simulink model "ovap_sim"  (R2025a)
settings: Solver=ode4  StartTime=0.0  StopTime=20  FixedStep=0.002  RelTol=1e-3
undefined symbols (not defined in the file): X, Y, Z
libraries: sm_lib x173, nesl_utility x72, simulink_extras x37, slpidlib x16, fl_lib x2
(part 4 of 5)

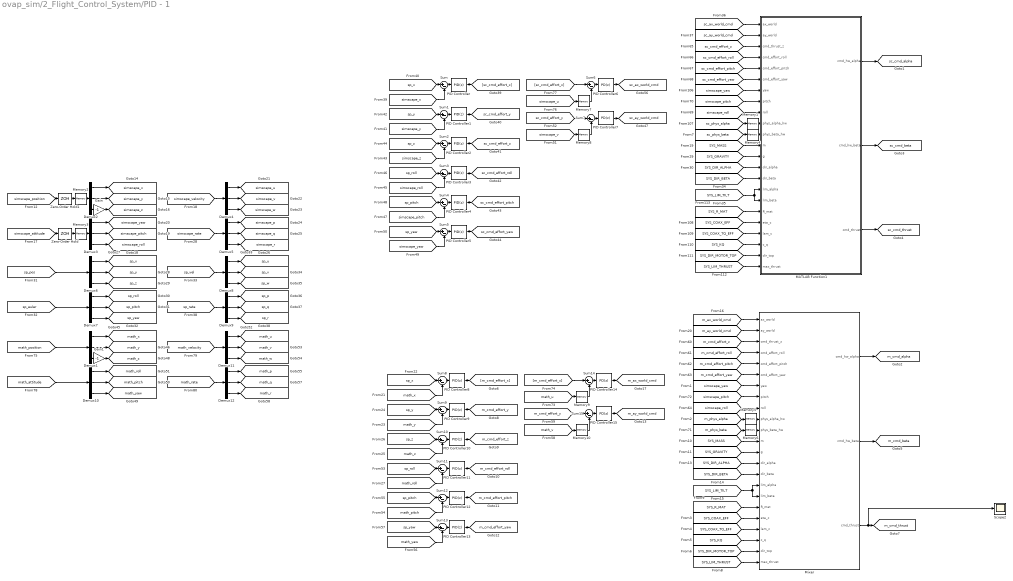
== system ovap_sim/2_Flight_Control_System/PID - 1 ==
  Demux{1..12} (12 alike) : Demux  Outputs=3
  Gain : Gain  Gain=-1
  Gain1 : Gain  Gain=-1
  MATLAB Function1 : MATLAB Function  TreatAsAtomicUnit=on
  Memory{1..10} (10 alike) : Memory
  Mixer : MATLAB Function  TreatAsAtomicUnit=on
  PID Controller : slpidlib/PID Controller  Controller=PID  Form=Parallel  TimeDomain=Discrete-time  UseExternalTs=off  SampleTime=0.002  IntegratorMethod=Forward Euler  FilterMethod=Forward Euler  ControllerParametersSource=internal  P=1  I=0  UseKiTs=off  D=0  UseExternalDerivativeSource=off  N=100  UseFilter=on  TunerSelectOption=Transfer Function Based (PID Tuner App)  InitialConditionSource=internal  InitialConditionForIntegrator=0  InitialConditionForFilter=0  DifferentiatorICPrevScaledInput=0  ExternalReset=none  TrackingMode=off  Kt=1  LimitOutput=off  SatLimitsSource=internal  UpperSaturationLimit=1  LowerSaturationLimit=-1  LinearizeAsGain=off  AntiWindupMode=clamping  Kb=1  LimitIntegrator=off  UpperIntegratorSaturationLimit=inf  LowerIntegratorSaturationLimit=-inf  POutMin=[]  POutMax=[]  IOutMin=[]  IOutMax=[]  DOutMin=[]  DOutMax=[]  NOutMin=[]  NOutMax=[]  SumOutMin=[]  SumOutMax=[]  SaturationOutMin=[]  SaturationOutMax=[]  PParamMin=[]  PParamMax=[]  IParamMin=[]  IParamMax=[]  DParamMin=[]  DParamMax=[]  NParamMin=[]  NParamMax=[]  KbParamMin=[]  KbParamMax=[]  KtParamMin=[]  KtParamMax=[]  KbOutMin=[]  KbOutMax=[]  KtOutMin=[]  KtOutMax=[]  IntegratorOutMin=[]  IntegratorOutMax=[]  FilterOutMin=[]  FilterOutMax=[]  SumI1OutMin=[]  SumI1OutMax=[]  SumI2OutMin=[]  SumI2OutMax=[]  SumI3OutMin=[]  SumI3OutMax=[]  SumI4OutMin=[]  SumI4OutMax=[]  SumDOutMin=[]  SumDOutMax=[]  DifferentiatorOutMin=[]  DifferentiatorOutMax=[]  FilterDiffOutCoefMin=[]  FilterDiffOutCoefMax=[]  ReciprocalOutMin=[]  ReciprocalOutMax=[]  SumDenOutMin=[]  SumDenOutMax=[]  SumNumOutMin=[]  SumNumOutMax=[]  DivideOutMin=[]  DivideOutMax=[]  UdiffTsProdOutMin=[]  UdiffTsProdOutMax=[]  NTsProdOutMin=[]  NTsProdOutMax=[]  UintegralTsProdOutMin=[]  UintegralTsProdOutMax=[]  UngainTsProdOutMin=[]  UngainTsProdOutMax=[]  ClampingZeroOutDataTypeStr=Inherit: Inherit via back propagation  ClampingZeroOutMin=[]  ClampingZeroOutMax=[]  FilterDenConstantOutDataTypeStr=Inherit: Inherit via back propagation  FilterDenConstantOutMin=[]  FilterDenConstantOutMax=[]  PCopyOutDataTypeStr=Inherit: Inherit via back propagation  PCopyOutMin=[]  PCopyOutMax=[]  NCopyOutDataTypeStr=Inherit: Inherit via back propagation  NCopyOutMin=[]  NCopyOutMax=[]  IntegratorContinuousStateAttributes=''  IntegratorStateMustResolveToSignalObject=off  IntegratorRTWStateStorageClass=Auto  FilterContinuousStateAttributes=''  FilterStateMustResolveToSignalObject=off  FilterRTWStateStorageClass=Auto  ParallelPVariant=InternalParameters  IdealPVariant=Disabled  IVariant=InternalParameters  DVariant=InternalParameters  IntegratorVariant=Discrete  SatVariant=Disabled  AWVariant=Passthrough  PCopyVariant=Disabled  TRVariant=Disabled  FdbkBlocksVariant=Forward  IdealPFdbkVariant=Disabled  SatFdbkVariant=Disabled  DerivativeFilterVariant=ForwardEulerFilter  NVariant=InternalParameters  NCopyVariant=Disabled  FilterICVariant=InternalICsFilter  IntegratorICVariant=InternalICs  ExternalResetVariant=Disabled  TRSumVariant=Passthrough  SumFdbkVariant=Disabled  SumVariant=Sum_PID  TsampFilterVariant=InternalTs  TsampNgainVariant=Passthrough  TsampIntegralVariant=Disabled_SignalSpec  ExternalSaturationOutDataTypeStr=Inherit: Same as second input  DerivativeSourceVariant=ErrorSignal  PreIntVariant=InternalPreInt
  PID Controller1 : slpidlib/PID Controller  Controller=PID  Form=Parallel  TimeDomain=Discrete-time  UseExternalTs=off  SampleTime=0.002  IntegratorMethod=Forward Euler  FilterMethod=Forward Euler  ControllerParametersSource=internal  P=1  I=0  UseKiTs=off  D=0  UseExternalDerivativeSource=off  N=100  UseFilter=on  TunerSelectOption=Transfer Function Based (PID Tuner App)  InitialConditionSource=internal  InitialConditionForIntegrator=0  InitialConditionForFilter=0  DifferentiatorICPrevScaledInput=0  ExternalReset=none  TrackingMode=off  Kt=1  LimitOutput=on  SatLimitsSource=internal  UpperSaturationLimit=5  LowerSaturationLimit=-5  LinearizeAsGain=on  AntiWindupMode=clamping  Kb=1  LimitIntegrator=off  UpperIntegratorSaturationLimit=inf  LowerIntegratorSaturationLimit=-inf  POutMin=[]  POutMax=[]  IOutMin=[]  IOutMax=[]  DOutMin=[]  DOutMax=[]  NOutMin=[]  NOutMax=[]  SumOutMin=[]  SumOutMax=[]  SaturationOutMin=[]  SaturationOutMax=[]  PParamMin=[]  PParamMax=[]  IParamMin=[]  IParamMax=[]  DParamMin=[]  DParamMax=[]  NParamMin=[]  NParamMax=[]  KbParamMin=[]  KbParamMax=[]  KtParamMin=[]  KtParamMax=[]  KbOutMin=[]  KbOutMax=[]  KtOutMin=[]  KtOutMax=[]  IntegratorOutMin=[]  IntegratorOutMax=[]  FilterOutMin=[]  FilterOutMax=[]  SumI1OutMin=[]  SumI1OutMax=[]  SumI2OutMin=[]  SumI2OutMax=[]  SumI3OutMin=[]  SumI3OutMax=[]  SumI4OutMin=[]  SumI4OutMax=[]  SumDOutMin=[]  SumDOutMax=[]  DifferentiatorOutMin=[]  DifferentiatorOutMax=[]  FilterDiffOutCoefMin=[]  FilterDiffOutCoefMax=[]  ReciprocalOutMin=[]  ReciprocalOutMax=[]  SumDenOutMin=[]  SumDenOutMax=[]  SumNumOutMin=[]  SumNumOutMax=[]  DivideOutMin=[]  DivideOutMax=[]  UdiffTsProdOutMin=[]  UdiffTsProdOutMax=[]  NTsProdOutMin=[]  NTsProdOutMax=[]  UintegralTsProdOutMin=[]  UintegralTsProdOutMax=[]  UngainTsProdOutMin=[]  UngainTsProdOutMax=[]  ClampingZeroOutDataTypeStr=Inherit: Inherit via back propagation  ClampingZeroOutMin=[]  ClampingZeroOutMax=[]  FilterDenConstantOutDataTypeStr=Inherit: Inherit via back propagation  FilterDenConstantOutMin=[]  FilterDenConstantOutMax=[]  PCopyOutDataTypeStr=Inherit: Inherit via back propagation  PCopyOutMin=[]  PCopyOutMax=[]  NCopyOutDataTypeStr=Inherit: Inherit via back propagation  NCopyOutMin=[]  NCopyOutMax=[]  IntegratorContinuousStateAttributes=''  IntegratorStateMustResolveToSignalObject=off  IntegratorRTWStateStorageClass=Auto  FilterContinuousStateAttributes=''  FilterStateMustResolveToSignalObject=off  FilterRTWStateStorageClass=Auto  ParallelPVariant=InternalParameters  IdealPVariant=Disabled  IVariant=InternalParameters  DVariant=InternalParameters  IntegratorVariant=Discrete  SatVariant=Enabled  AWVariant=DiscClampingParallel  PCopyVariant=Disabled  TRVariant=Disabled  FdbkBlocksVariant=Forward  IdealPFdbkVariant=Disabled  SatFdbkVariant=Disabled  DerivativeFilterVariant=ForwardEulerFilter  NVariant=InternalParameters  NCopyVariant=Disabled  FilterICVariant=InternalICsFilter  IntegratorICVariant=InternalICs  ExternalResetVariant=Disabled  TRSumVariant=Passthrough  SumFdbkVariant=Disabled  SumVariant=Sum_PID  TsampFilterVariant=InternalTs  TsampNgainVariant=Passthrough  TsampIntegralVariant=Disabled_SignalSpec  ExternalSaturationOutDataTypeStr=Inherit: Same as second input  DerivativeSourceVariant=ErrorSignal  PreIntVariant=InternalPreInt
  PID Controller10 : slpidlib/PID Controller  Controller=PID  Form=Parallel  TimeDomain=Discrete-time  UseExternalTs=off  SampleTime=0.002  IntegratorMethod=Forward Euler  FilterMethod=Forward Euler  ControllerParametersSource=internal  P=2  I=0.0001  UseKiTs=off  D=4  UseExternalDerivativeSource=off  N=100  UseFilter=on  TunerSelectOption=Transfer Function Based (PID Tuner App)  InitialConditionSource=internal  InitialConditionForIntegrator=0  InitialConditionForFilter=0  DifferentiatorICPrevScaledInput=0  ExternalReset=none  TrackingMode=off  Kt=1  LimitOutput=on  SatLimitsSource=internal  UpperSaturationLimit=5  LowerSaturationLimit=-5  LinearizeAsGain=on  AntiWindupMode=clamping  Kb=1  LimitIntegrator=off  UpperIntegratorSaturationLimit=inf  LowerIntegratorSaturationLimit=-inf  POutMin=[]  POutMax=[]  IOutMin=[]  IOutMax=[]  DOutMin=[]  DOutMax=[]  NOutMin=[]  NOutMax=[]  SumOutMin=[]  SumOutMax=[]  SaturationOutMin=[]  SaturationOutMax=[]  PParamMin=[]  PParamMax=[]  IParamMin=[]  IParamMax=[]  DParamMin=[]  DParamMax=[]  NParamMin=[]  NParamMax=[]  KbParamMin=[]  KbParamMax=[]  KtParamMin=[]  KtParamMax=[]  KbOutMin=[]  KbOutMax=[]  KtOutMin=[]  KtOutMax=[]  IntegratorOutMin=[]  IntegratorOutMax=[]  FilterOutMin=[]  FilterOutMax=[]  SumI1OutMin=[]  SumI1OutMax=[]  SumI2OutMin=[]  SumI2OutMax=[]  SumI3OutMin=[]  SumI3OutMax=[]  SumI4OutMin=[]  SumI4OutMax=[]  SumDOutMin=[]  SumDOutMax=[]  DifferentiatorOutMin=[]  DifferentiatorOutMax=[]  FilterDiffOutCoefMin=[]  FilterDiffOutCoefMax=[]  ReciprocalOutMin=[]  ReciprocalOutMax=[]  SumDenOutMin=[]  SumDenOutMax=[]  SumNumOutMin=[]  SumNumOutMax=[]  DivideOutMin=[]  DivideOutMax=[]  UdiffTsProdOutMin=[]  UdiffTsProdOutMax=[]  NTsProdOutMin=[]  NTsProdOutMax=[]  UintegralTsProdOutMin=[]  UintegralTsProdOutMax=[]  UngainTsProdOutMin=[]  UngainTsProdOutMax=[]  ClampingZeroOutDataTypeStr=Inherit: Inherit via back propagation  ClampingZeroOutMin=[]  ClampingZeroOutMax=[]  FilterDenConstantOutDataTypeStr=Inherit: Inherit via back propagation  FilterDenConstantOutMin=[]  FilterDenConstantOutMax=[]  PCopyOutDataTypeStr=Inherit: Inherit via back propagation  PCopyOutMin=[]  PCopyOutMax=[]  NCopyOutDataTypeStr=Inherit: Inherit via back propagation  NCopyOutMin=[]  NCopyOutMax=[]  IntegratorContinuousStateAttributes=''  IntegratorStateMustResolveToSignalObject=off  IntegratorRTWStateStorageClass=Auto  FilterContinuousStateAttributes=''  FilterStateMustResolveToSignalObject=off  FilterRTWStateStorageClass=Auto  ParallelPVariant=InternalParameters  IdealPVariant=Disabled  IVariant=InternalParameters  DVariant=InternalParameters  IntegratorVariant=Discrete  SatVariant=Enabled  AWVariant=DiscClampingParallel  PCopyVariant=Disabled  TRVariant=Disabled  FdbkBlocksVariant=Forward  IdealPFdbkVariant=Disabled  SatFdbkVariant=Disabled  DerivativeFilterVariant=ForwardEulerFilter  NVariant=InternalParameters  NCopyVariant=Disabled  FilterICVariant=InternalICsFilter  IntegratorICVariant=InternalICs  ExternalResetVariant=Disabled  TRSumVariant=Passthrough  SumFdbkVariant=Disabled  SumVariant=Sum_PID  TsampFilterVariant=InternalTs  TsampNgainVariant=Passthrough  TsampIntegralVariant=Disabled_SignalSpec  ExternalSaturationOutDataTypeStr=Inherit: Same as second input  DerivativeSourceVariant=ErrorSignal  PreIntVariant=InternalPreInt
  PID Controller{3..5,11..13} (6 alike) : slpidlib/PID Controller  Controller=PID  Form=Parallel  TimeDomain=Discrete-time  UseExternalTs=off  SampleTime=0.002  IntegratorMethod=Forward Euler  FilterMethod=Forward Euler  ControllerParametersSource=internal  P=1  I=0  UseKiTs=off  D=0  UseExternalDerivativeSource=off  N=100  UseFilter=on  TunerSelectOption=Transfer Function Based (PID Tuner App)  InitialConditionSource=internal  InitialConditionForIntegrator=0  InitialConditionForFilter=0  DifferentiatorICPrevScaledInput=0  ExternalReset=none  TrackingMode=off  Kt=1  LimitOutput=on  SatLimitsSource=internal  UpperSaturationLimit=5  LowerSaturationLimit=-5  LinearizeAsGain=on  AntiWindupMode=none  Kb=1  LimitIntegrator=off  UpperIntegratorSaturationLimit=inf  LowerIntegratorSaturationLimit=-inf  POutMin=[]  POutMax=[]  IOutMin=[]  IOutMax=[]  DOutMin=[]  DOutMax=[]  NOutMin=[]  NOutMax=[]  SumOutMin=[]  SumOutMax=[]  SaturationOutMin=[]  SaturationOutMax=[]  PParamMin=[]  PParamMax=[]  IParamMin=[]  IParamMax=[]  DParamMin=[]  DParamMax=[]  NParamMin=[]  NParamMax=[]  KbParamMin=[]  KbParamMax=[]  KtParamMin=[]  KtParamMax=[]  KbOutMin=[]  KbOutMax=[]  KtOutMin=[]  KtOutMax=[]  IntegratorOutMin=[]  IntegratorOutMax=[]  FilterOutMin=[]  FilterOutMax=[]  SumI1OutMin=[]  SumI1OutMax=[]  SumI2OutMin=[]  SumI2OutMax=[]  SumI3OutMin=[]  SumI3OutMax=[]  SumI4OutMin=[]  SumI4OutMax=[]  SumDOutMin=[]  SumDOutMax=[]  DifferentiatorOutMin=[]  DifferentiatorOutMax=[]  FilterDiffOutCoefMin=[]  FilterDiffOutCoefMax=[]  ReciprocalOutMin=[]  ReciprocalOutMax=[]  SumDenOutMin=[]  SumDenOutMax=[]  SumNumOutMin=[]  SumNumOutMax=[]  DivideOutMin=[]  DivideOutMax=[]  UdiffTsProdOutMin=[]  UdiffTsProdOutMax=[]  NTsProdOutMin=[]  NTsProdOutMax=[]  UintegralTsProdOutMin=[]  UintegralTsProdOutMax=[]  UngainTsProdOutMin=[]  UngainTsProdOutMax=[]  ClampingZeroOutDataTypeStr=Inherit: Inherit via back propagation  ClampingZeroOutMin=[]  ClampingZeroOutMax=[]  FilterDenConstantOutDataTypeStr=Inherit: Inherit via back propagation  FilterDenConstantOutMin=[]  FilterDenConstantOutMax=[]  PCopyOutDataTypeStr=Inherit: Inherit via back propagation  PCopyOutMin=[]  PCopyOutMax=[]  NCopyOutDataTypeStr=Inherit: Inherit via back propagation  NCopyOutMin=[]  NCopyOutMax=[]  IntegratorContinuousStateAttributes=''  IntegratorStateMustResolveToSignalObject=off  IntegratorRTWStateStorageClass=Auto  FilterContinuousStateAttributes=''  FilterStateMustResolveToSignalObject=off  FilterRTWStateStorageClass=Auto  ParallelPVariant=InternalParameters  IdealPVariant=Disabled  IVariant=InternalParameters  DVariant=InternalParameters  IntegratorVariant=Discrete  SatVariant=Enabled  AWVariant=Passthrough  PCopyVariant=Disabled  TRVariant=Disabled  FdbkBlocksVariant=Forward  IdealPFdbkVariant=Disabled  SatFdbkVariant=Disabled  DerivativeFilterVariant=ForwardEulerFilter  NVariant=InternalParameters  NCopyVariant=Disabled  FilterICVariant=InternalICsFilter  IntegratorICVariant=InternalICs  ExternalResetVariant=Disabled  TRSumVariant=Passthrough  SumFdbkVariant=Disabled  SumVariant=Sum_PID  TsampFilterVariant=InternalTs  TsampNgainVariant=Passthrough  TsampIntegralVariant=Disabled_SignalSpec  ExternalSaturationOutDataTypeStr=Inherit: Same as second input  DerivativeSourceVariant=ErrorSignal  PreIntVariant=InternalPreInt
  PID Controller{6..7,14..15} (4 alike) : slpidlib/PID Controller  Controller=PD  Form=Parallel  TimeDomain=Discrete-time  UseExternalTs=off  SampleTime=0.002  IntegratorMethod=Forward Euler  FilterMethod=Forward Euler  ControllerParametersSource=internal  P=1  I=0  UseKiTs=off  D=0  UseExternalDerivativeSource=off  N=100  UseFilter=on  TunerSelectOption=Transfer Function Based (PID Tuner App)  InitialConditionSource=internal  InitialConditionForIntegrator=0  InitialConditionForFilter=0  DifferentiatorICPrevScaledInput=0  ExternalReset=none  TrackingMode=off  Kt=1  LimitOutput=on  SatLimitsSource=internal  UpperSaturationLimit=3  LowerSaturationLimit=-3  LinearizeAsGain=off  AntiWindupMode=clamping  Kb=1  LimitIntegrator=off  UpperIntegratorSaturationLimit=inf  LowerIntegratorSaturationLimit=-inf  POutMin=[]  POutMax=[]  IOutMin=[]  IOutMax=[]  DOutMin=[]  DOutMax=[]  NOutMin=[]  NOutMax=[]  SumOutMin=[]  SumOutMax=[]  SaturationOutMin=[]  SaturationOutMax=[]  PParamMin=[]  PParamMax=[]  IParamMin=[]  IParamMax=[]  DParamMin=[]  DParamMax=[]  NParamMin=[]  NParamMax=[]  KbParamMin=[]  KbParamMax=[]  KtParamMin=[]  KtParamMax=[]  KbOutMin=[]  KbOutMax=[]  KtOutMin=[]  KtOutMax=[]  IntegratorOutMin=[]  IntegratorOutMax=[]  FilterOutMin=[]  FilterOutMax=[]  SumI1OutMin=[]  SumI1OutMax=[]  SumI2OutMin=[]  SumI2OutMax=[]  SumI3OutMin=[]  SumI3OutMax=[]  SumI4OutMin=[]  SumI4OutMax=[]  SumDOutMin=[]  SumDOutMax=[]  DifferentiatorOutMin=[]  DifferentiatorOutMax=[]  FilterDiffOutCoefMin=[]  FilterDiffOutCoefMax=[]  ReciprocalOutMin=[]  ReciprocalOutMax=[]  SumDenOutMin=[]  SumDenOutMax=[]  SumNumOutMin=[]  SumNumOutMax=[]  DivideOutMin=[]  DivideOutMax=[]  UdiffTsProdOutMin=[]  UdiffTsProdOutMax=[]  NTsProdOutMin=[]  NTsProdOutMax=[]  UintegralTsProdOutMin=[]  UintegralTsProdOutMax=[]  UngainTsProdOutMin=[]  UngainTsProdOutMax=[]  ClampingZeroOutDataTypeStr=Inherit: Inherit via back propagation  ClampingZeroOutMin=[]  ClampingZeroOutMax=[]  FilterDenConstantOutDataTypeStr=Inherit: Inherit via back propagation  FilterDenConstantOutMin=[]  FilterDenConstantOutMax=[]  PCopyOutDataTypeStr=Inherit: Inherit via back propagation  PCopyOutMin=[]  PCopyOutMax=[]  NCopyOutDataTypeStr=Inherit: Inherit via back propagation  NCopyOutMin=[]  NCopyOutMax=[]  IntegratorContinuousStateAttributes=''  IntegratorStateMustResolveToSignalObject=off  IntegratorRTWStateStorageClass=Auto  FilterContinuousStateAttributes=''  FilterStateMustResolveToSignalObject=off  FilterRTWStateStorageClass=Auto  ParallelPVariant=InternalParameters  IdealPVariant=Disabled  IVariant=Disabled  DVariant=InternalParameters  IntegratorVariant=Disabled  SatVariant=Enabled  AWVariant=Disabled  PCopyVariant=Disabled  TRVariant=Disabled  FdbkBlocksVariant=Forward  IdealPFdbkVariant=Disabled  SatFdbkVariant=Disabled  DerivativeFilterVariant=ForwardEulerFilter  NVariant=InternalParameters  NCopyVariant=Disabled  FilterICVariant=InternalICsFilter  IntegratorICVariant=Disabled  ExternalResetVariant=Disabled  TRSumVariant=Passthrough  SumFdbkVariant=Disabled  SumVariant=Sum_PD  TsampFilterVariant=InternalTs  TsampNgainVariant=Passthrough  TsampIntegralVariant=Disabled_SignalSpec  ExternalSaturationOutDataTypeStr=Inherit: Same as second input  DerivativeSourceVariant=ErrorSignal  PreIntVariant=InternalPreInt
  PID Controller2 : slpidlib/PID Controller  Controller=PID  Form=Parallel  TimeDomain=Discrete-time  UseExternalTs=off  SampleTime=0.002  IntegratorMethod=Forward Euler  FilterMethod=Forward Euler  ControllerParametersSource=internal  P=2  I=0.0001  UseKiTs=off  D=4.2  UseExternalDerivativeSource=off  N=100  UseFilter=on  TunerSelectOption=Transfer Function Based (PID Tuner App)  InitialConditionSource=internal  InitialConditionForIntegrator=0  InitialConditionForFilter=0  DifferentiatorICPrevScaledInput=0  ExternalReset=none  TrackingMode=off  Kt=1  LimitOutput=on  SatLimitsSource=internal  UpperSaturationLimit=5  LowerSaturationLimit=-5  LinearizeAsGain=on  AntiWindupMode=clamping  Kb=1  LimitIntegrator=off  UpperIntegratorSaturationLimit=inf  LowerIntegratorSaturationLimit=-inf  POutMin=[]  POutMax=[]  IOutMin=[]  IOutMax=[]  DOutMin=[]  DOutMax=[]  NOutMin=[]  NOutMax=[]  SumOutMin=[]  SumOutMax=[]  SaturationOutMin=[]  SaturationOutMax=[]  PParamMin=[]  PParamMax=[]  IParamMin=[]  IParamMax=[]  DParamMin=[]  DParamMax=[]  NParamMin=[]  NParamMax=[]  KbParamMin=[]  KbParamMax=[]  KtParamMin=[]  KtParamMax=[]  KbOutMin=[]  KbOutMax=[]  KtOutMin=[]  KtOutMax=[]  IntegratorOutMin=[]  IntegratorOutMax=[]  FilterOutMin=[]  FilterOutMax=[]  SumI1OutMin=[]  SumI1OutMax=[]  SumI2OutMin=[]  SumI2OutMax=[]  SumI3OutMin=[]  SumI3OutMax=[]  SumI4OutMin=[]  SumI4OutMax=[]  SumDOutMin=[]  SumDOutMax=[]  DifferentiatorOutMin=[]  DifferentiatorOutMax=[]  FilterDiffOutCoefMin=[]  FilterDiffOutCoefMax=[]  ReciprocalOutMin=[]  ReciprocalOutMax=[]  SumDenOutMin=[]  SumDenOutMax=[]  SumNumOutMin=[]  SumNumOutMax=[]  DivideOutMin=[]  DivideOutMax=[]  UdiffTsProdOutMin=[]  UdiffTsProdOutMax=[]  NTsProdOutMin=[]  NTsProdOutMax=[]  UintegralTsProdOutMin=[]  UintegralTsProdOutMax=[]  UngainTsProdOutMin=[]  UngainTsProdOutMax=[]  ClampingZeroOutDataTypeStr=Inherit: Inherit via back propagation  ClampingZeroOutMin=[]  ClampingZeroOutMax=[]  FilterDenConstantOutDataTypeStr=Inherit: Inherit via back propagation  FilterDenConstantOutMin=[]  FilterDenConstantOutMax=[]  PCopyOutDataTypeStr=Inherit: Inherit via back propagation  PCopyOutMin=[]  PCopyOutMax=[]  NCopyOutDataTypeStr=Inherit: Inherit via back propagation  NCopyOutMin=[]  NCopyOutMax=[]  IntegratorContinuousStateAttributes=''  IntegratorStateMustResolveToSignalObject=off  IntegratorRTWStateStorageClass=Auto  FilterContinuousStateAttributes=''  FilterStateMustResolveToSignalObject=off  FilterRTWStateStorageClass=Auto  ParallelPVariant=InternalParameters  IdealPVariant=Disabled  IVariant=InternalParameters  DVariant=InternalParameters  IntegratorVariant=Discrete  SatVariant=Enabled  AWVariant=DiscClampingParallel  PCopyVariant=Disabled  TRVariant=Disabled  FdbkBlocksVariant=Forward  IdealPFdbkVariant=Disabled  SatFdbkVariant=Disabled  DerivativeFilterVariant=ForwardEulerFilter  NVariant=InternalParameters  NCopyVariant=Disabled  FilterICVariant=InternalICsFilter  IntegratorICVariant=InternalICs  ExternalResetVariant=Disabled  TRSumVariant=Passthrough  SumFdbkVariant=Disabled  SumVariant=Sum_PID  TsampFilterVariant=InternalTs  TsampNgainVariant=Passthrough  TsampIntegralVariant=Disabled_SignalSpec  ExternalSaturationOutDataTypeStr=Inherit: Same as second input  DerivativeSourceVariant=ErrorSignal  PreIntVariant=InternalPreInt
  PID Controller8 : slpidlib/PID Controller  Controller=PID  Form=Parallel  TimeDomain=Discrete-time  UseExternalTs=off  SampleTime=0.002  IntegratorMethod=Forward Euler  FilterMethod=Forward Euler  ControllerParametersSource=internal  P=1  I=0  UseKiTs=off  D=0  UseExternalDerivativeSource=off  N=100  UseFilter=on  TunerSelectOption=Transfer Function Based (PID Tuner App)  InitialConditionSource=internal  InitialConditionForIntegrator=0  InitialConditionForFilter=0  DifferentiatorICPrevScaledInput=0  ExternalReset=none  TrackingMode=off  Kt=1  LimitOutput=off  SatLimitsSource=internal  UpperSaturationLimit=1  LowerSaturationLimit=-1  LinearizeAsGain=off  AntiWindupMode=clamping  Kb=1  LimitIntegrator=off  UpperIntegratorSaturationLimit=inf  LowerIntegratorSaturationLimit=-inf  POutMin=[]  POutMax=[]  IOutMin=[]  IOutMax=[]  DOutMin=[]  DOutMax=[]  NOutMin=[]  NOutMax=[]  SumOutMin=[]  SumOutMax=[]  SaturationOutMin=[]  SaturationOutMax=[]  PParamMin=[]  PParamMax=[]  IParamMin=[]  IParamMax=[]  DParamMin=[]  DParamMax=[]  NParamMin=[]  NParamMax=[]  KbParamMin=[]  KbParamMax=[]  KtParamMin=[]  KtParamMax=[]  KbOutMin=[]  KbOutMax=[]  KtOutMin=[]  KtOutMax=[]  IntegratorOutMin=[]  IntegratorOutMax=[]  FilterOutMin=[]  FilterOutMax=[]  SumI1OutMin=[]  SumI1OutMax=[]  SumI2OutMin=[]  SumI2OutMax=[]  SumI3OutMin=[]  SumI3OutMax=[]  SumI4OutMin=[]  SumI4OutMax=[]  SumDOutMin=[]  SumDOutMax=[]  DifferentiatorOutMin=[]  DifferentiatorOutMax=[]  FilterDiffOutCoefMin=[]  FilterDiffOutCoefMax=[]  ReciprocalOutMin=[]  ReciprocalOutMax=[]  SumDenOutMin=[]  SumDenOutMax=[]  SumNumOutMin=[]  SumNumOutMax=[]  DivideOutMin=[]  DivideOutMax=[]  UdiffTsProdOutMin=[]  UdiffTsProdOutMax=[]  NTsProdOutMin=[]  NTsProdOutMax=[]  UintegralTsProdOutMin=[]  UintegralTsProdOutMax=[]  UngainTsProdOutMin=[]  UngainTsProdOutMax=[]  ClampingZeroOutDataTypeStr=Inherit: Inherit via back propagation  ClampingZeroOutMin=[]  ClampingZeroOutMax=[]  FilterDenConstantOutDataTypeStr=Inherit: Inherit via back propagation  FilterDenConstantOutMin=[]  FilterDenConstantOutMax=[]  PCopyOutDataTypeStr=Inherit: Inherit via back propagation  PCopyOutMin=[]  PCopyOutMax=[]  NCopyOutDataTypeStr=Inherit: Inherit via back propagation  NCopyOutMin=[]  NCopyOutMax=[]  IntegratorContinuousStateAttributes=''  IntegratorStateMustResolveToSignalObject=off  IntegratorRTWStateStorageClass=Auto  FilterContinuousStateAttributes=''  FilterStateMustResolveToSignalObject=off  FilterRTWStateStorageClass=Auto  ParallelPVariant=InternalParameters  IdealPVariant=Disabled  IVariant=InternalParameters  DVariant=InternalParameters  IntegratorVariant=Discrete  SatVariant=Disabled  AWVariant=Passthrough  PCopyVariant=Disabled  TRVariant=Disabled  FdbkBlocksVariant=Forward  IdealPFdbkVariant=Disabled  SatFdbkVariant=Disabled  DerivativeFilterVariant=ForwardEulerFilter  NVariant=InternalParameters  NCopyVariant=Disabled  FilterICVariant=InternalICsFilter  IntegratorICVariant=InternalICs  ExternalResetVariant=Disabled  TRSumVariant=Passthrough  SumFdbkVariant=Disabled  SumVariant=Sum_PID  TsampFilterVariant=InternalTs  TsampNgainVariant=Passthrough  TsampIntegralVariant=Disabled_SignalSpec  ExternalSaturationOutDataTypeStr=Inherit: Same as second input  DerivativeSourceVariant=ErrorSignal  PreIntVariant=InternalPreInt
  PID Controller9 : slpidlib/PID Controller  Controller=PID  Form=Parallel  TimeDomain=Discrete-time  UseExternalTs=off  SampleTime=0.002  IntegratorMethod=Forward Euler  FilterMethod=Forward Euler  ControllerParametersSource=internal  P=1  I=0  UseKiTs=off  D=0  UseExternalDerivativeSource=off  N=100  UseFilter=on  TunerSelectOption=Transfer Function Based (PID Tuner App)  InitialConditionSource=internal  InitialConditionForIntegrator=0  InitialConditionForFilter=0  DifferentiatorICPrevScaledInput=0  ExternalReset=none  TrackingMode=off  Kt=1  LimitOutput=on  SatLimitsSource=internal  UpperSaturationLimit=5  LowerSaturationLimit=-5  LinearizeAsGain=on  AntiWindupMode=clamping  Kb=1  LimitIntegrator=off  UpperIntegratorSaturationLimit=inf  LowerIntegratorSaturationLimit=-inf  POutMin=[]  POutMax=[]  IOutMin=[]  IOutMax=[]  DOutMin=[]  DOutMax=[]  NOutMin=[]  NOutMax=[]  SumOutMin=[]  SumOutMax=[]  SaturationOutMin=[]  SaturationOutMax=[]  PParamMin=[]  PParamMax=[]  IParamMin=[]  IParamMax=[]  DParamMin=[]  DParamMax=[]  NParamMin=[]  NParamMax=[]  KbParamMin=[]  KbParamMax=[]  KtParamMin=[]  KtParamMax=[]  KbOutMin=[]  KbOutMax=[]  KtOutMin=[]  KtOutMax=[]  IntegratorOutMin=[]  IntegratorOutMax=[]  FilterOutMin=[]  FilterOutMax=[]  SumI1OutMin=[]  SumI1OutMax=[]  SumI2OutMin=[]  SumI2OutMax=[]  SumI3OutMin=[]  SumI3OutMax=[]  SumI4OutMin=[]  SumI4OutMax=[]  SumDOutMin=[]  SumDOutMax=[]  DifferentiatorOutMin=[]  DifferentiatorOutMax=[]  FilterDiffOutCoefMin=[]  FilterDiffOutCoefMax=[]  ReciprocalOutMin=[]  ReciprocalOutMax=[]  SumDenOutMin=[]  SumDenOutMax=[]  SumNumOutMin=[]  SumNumOutMax=[]  DivideOutMin=[]  DivideOutMax=[]  UdiffTsProdOutMin=[]  UdiffTsProdOutMax=[]  NTsProdOutMin=[]  NTsProdOutMax=[]  UintegralTsProdOutMin=[]  UintegralTsProdOutMax=[]  UngainTsProdOutMin=[]  UngainTsProdOutMax=[]  ClampingZeroOutDataTypeStr=Inherit: Inherit via back propagation  ClampingZeroOutMin=[]  ClampingZeroOutMax=[]  FilterDenConstantOutDataTypeStr=Inherit: Inherit via back propagation  FilterDenConstantOutMin=[]  FilterDenConstantOutMax=[]  PCopyOutDataTypeStr=Inherit: Inherit via back propagation  PCopyOutMin=[]  PCopyOutMax=[]  NCopyOutDataTypeStr=Inherit: Inherit via back propagation  NCopyOutMin=[]  NCopyOutMax=[]  IntegratorContinuousStateAttributes=''  IntegratorStateMustResolveToSignalObject=off  IntegratorRTWStateStorageClass=Auto  FilterContinuousStateAttributes=''  FilterStateMustResolveToSignalObject=off  FilterRTWStateStorageClass=Auto  ParallelPVariant=InternalParameters  IdealPVariant=Disabled  IVariant=InternalParameters  DVariant=InternalParameters  IntegratorVariant=Discrete  SatVariant=Enabled  AWVariant=DiscClampingParallel  PCopyVariant=Disabled  TRVariant=Disabled  FdbkBlocksVariant=Forward  IdealPFdbkVariant=Disabled  SatFdbkVariant=Disabled  DerivativeFilterVariant=ForwardEulerFilter  NVariant=InternalParameters  NCopyVariant=Disabled  FilterICVariant=InternalICsFilter  IntegratorICVariant=InternalICs  ExternalResetVariant=Disabled  TRSumVariant=Passthrough  SumFdbkVariant=Disabled  SumVariant=Sum_PID  TsampFilterVariant=InternalTs  TsampNgainVariant=Passthrough  TsampIntegralVariant=Disabled_SignalSpec  ExternalSaturationOutDataTypeStr=Inherit: Same as second input  DerivativeSourceVariant=ErrorSignal  PreIntVariant=InternalPreInt
  Scope2 : Scope
      settings: ActiveDisplayYMinimum=2.634685350754407  ActiveDisplayYMaximum=5.63815135293212  DataLoggingVariableName=ScopeData25
  Sum{,1..15} (16 alike) : Sum  Inputs=|+-
  Zero-Order Hold : ZeroOrderHold  SampleTime=0.002
  Zero-Order Hold1 : ZeroOrderHold  SampleTime=0.002
  tag scope: m_ax_world_cmd=global, m_ay_world_cmd=global, m_cmd_alpha=global, m_cmd_beta=global, m_cmd_effort_pitch=global, m_cmd_effort_roll=global, m_cmd_effort_y=global, m_cmd_effort_yaw=global, m_cmd_effort_z=global, m_cmd_thrust=global, math_p=global, math_pitch=global, math_q=global, math_r=global, math_roll=global, math_u=global, math_v=global, math_w=global, math_x=global, math_y=global, math_yaw=global, math_z=global, sc_ax_world_cmd=global, sc_ay_world_cmd=global, sc_cmd_alpha=global, sc_cmd_beta=global, sc_cmd_effort_pitch=global, sc_cmd_effort_roll=global, sc_cmd_effort_y=global, sc_cmd_effort_yaw=global, sc_cmd_effort_z=global, sc_cmd_thrust=global, simscape_p=global, simscape_pitch=global, simscape_q=global, simscape_r=global, simscape_roll=global, simscape_u=global, simscape_v=global, simscape_w=global, simscape_x=global, simscape_y=global, simscape_yaw=global, simscape_z=global, sp_p=global, sp_pitch=global, sp_q=global, sp_r=global, sp_roll=global, sp_u=global, sp_v=global, sp_w=global, sp_x=global, sp_y=global, sp_yaw=global, sp_z=global
  wires:
  [simscape_position] -> Zero-Order Hold1/1
  Demux2/1 -> [simscape_x]
  Demux2/2 -> [simscape_y]
  [simscape_attitude] -> Zero-Order Hold/1
  [simscape_rate] -> Demux5/1
  Demux5/2 -> [simscape_q]
  Demux5/1 -> [simscape_p]
  Demux5/3 -> [simscape_r]
  Demux4/1 -> [simscape_u]
  [simscape_velocity] -> Demux4/1
  Demux4/2 -> [simscape_v]
  Demux4/3 -> [simscape_w]
  Demux7/1 -> [sp_roll]
  Demux7/3 -> [sp_yaw]
  Demux6/1 -> [sp_x]
  [sp_pos] -> Demux6/1
  Demux9/3 -> [sp_r]
  Demux9/1 -> [sp_p]
  Demux9/2 -> [sp_q]
  Demux8/2 -> [sp_v]
  Demux8/3 -> [sp_w]
  Demux8/1 -> [sp_u]
  [sp_vel] -> Demux8/1
  [sp_euler] -> Demux7/1
  Demux7/2 -> [sp_pitch]
  Demux6/2 -> [sp_y]
  Demux6/3 -> [sp_z]
  [sp_rate] -> Demux9/1
  [sp_x] -> Sum/1
  [simscape_x] -> Sum/2
  Sum/1 -> PID Controller/1
  PID Controller/1 -> [sc_cmd_effort_x]
  [simscape_y] -> Sum1/2
  Sum1/1 -> PID Controller1/1
  [sp_y] -> Sum1/1
  PID Controller1/1 -> [sc_cmd_effort_y]
  [simscape_z] -> Sum2/2
  Sum2/1 -> PID Controller2/1
  [sp_z] -> Sum2/1
  PID Controller3/1 -> [sc_cmd_effort_roll]
  [simscape_roll] -> Sum3/2
  PID Controller5/1 -> [sc_cmd_effort_yaw]
  [sp_yaw] -> Sum5/1
  [simscape_yaw] -> Sum5/2
  PID Controller4/1 -> [sc_cmd_effort_pitch]
  [sp_pitch] -> Sum4/1
  Sum4/1 -> PID Controller4/1
  Sum3/1 -> PID Controller3/1
  Sum5/1 -> PID Controller5/1
  [simscape_pitch] -> Sum4/2
  [sp_roll] -> Sum3/1
  Memory2/1 -> Demux2/1
  Memory3/1 -> Demux3/1
  Zero-Order Hold/1 -> Memory3/1
  Zero-Order Hold1/1 -> Memory2/1
  Demux2/3 -> Gain/1
  Gain/1 -> [simscape_z]
  Demux3/1 -> [simscape_yaw]
  Demux3/2 -> [simscape_pitch]
  Demux3/3 -> [simscape_roll]
  Sum6/1 -> PID Controller6/1
  [sc_cmd_effort_x] -> Sum6/1
  [simscape_u] -> Memory7/1
  [simscape_v] -> Memory8/1
  PID Controller7/1 -> [sc_ay_world_cmd]
  [sc_cmd_effort_y] -> Sum7/1
  Sum7/1 -> PID Controller7/1
  Memory7/1 -> Sum6/2
  Memory8/1 -> Sum7/2
  PID Controller6/1 -> [sc_ax_world_cmd]
  MATLAB Function1/1(cmd_hw_alpha) -> [sc_cmd_alpha]
  MATLAB Function1/2(cmd_hw_beta) -> [sc_cmd_beta]
  MATLAB Function1/3(cmd_thrust) -> [sc_cmd_thrust]
  [sc_ax_world_cmd] -> MATLAB Function1/1(ax_world)
  [sc_ay_world_cmd] -> MATLAB Function1/2(ay_world)
  [sc_cmd_effort_z] -> MATLAB Function1/3(cmd_thrust_z)
  [sc_cmd_effort_roll] -> MATLAB Function1/4(cmd_effort_roll)
  [sc_cmd_effort_pitch] -> MATLAB Function1/5(cmd_effort_pitch)
  [sc_cmd_effort_yaw] -> MATLAB Function1/6(cmd_effort_yaw)
  [simscape_yaw] -> MATLAB Function1/7(yaw)
  [simscape_pitch] -> MATLAB Function1/8(pitch)
  [simscape_roll] -> MATLAB Function1/9(roll)
  [SYS_MASS] -> MATLAB Function1/12(m)
  [SYS_GRAVITY] -> MATLAB Function1/13(g)
  [SYS_DIR_ALPHA] -> MATLAB Function1/14(dir_alpha)
  [SYS_DIR_BETA] -> MATLAB Function1/15(dir_beta)
  [SYS_LIM_TILT] -> MATLAB Function1/16(lim_alpha), MATLAB Function1/17(lim_beta)
  [SYS_COAX_EFF] -> MATLAB Function1/19(eta_c)
  [SYS_COAX_TQ_EFF] -> MATLAB Function1/20(lam_c)
  [SYS_KQ] -> MATLAB Function1/21(c_q)
  [SYS_DIR_MOTOR_TOP] -> MATLAB Function1/22(dir_top)
  [SYS_LIM_THRUST] -> MATLAB Function1/23(max_thrust)
  [SYS_R_MAT] -> MATLAB Function1/18(R_mat)
  Memory1/1 -> MATLAB Function1/10(phys_alpha_hw)
  [sc_phys_alpha] -> Memory1/1
  [sc_phys_beta] -> Memory4/1
  Memory4/1 -> MATLAB Function1/11(phys_beta_hw)
  PID Controller2/1 -> [sc_cmd_effort_z]
  [m_cmd_effort_roll] -> Mixer/4(cmd_effort_roll)
  [math_u] -> Memory9/1
  [SYS_LIM_TILT] -> Mixer/16(lim_alpha), Mixer/17(lim_beta)
  [simscape_pitch] -> Mixer/8(pitch)
  [SYS_R_MAT] -> Mixer/18(R_mat)
  Memory10/1 -> Sum15/2
  Sum14/1 -> PID Controller14/1
  [m_cmd_effort_x] -> Sum14/1
  [math_x] -> Sum8/2
  [m_phys_beta] -> Memory6/1
  [math_yaw] -> Sum13/2
  Mixer/2(cmd_hw_beta) -> [m_cmd_beta]
  [sp_yaw] -> Sum13/1
  [SYS_DIR_BETA] -> Mixer/15(dir_beta)
  Mixer/3(cmd_thrust) -> Scope2/1, [m_cmd_thrust]
  Sum10/1 -> PID Controller10/1
  PID Controller11/1 -> [m_cmd_effort_roll]
  [m_cmd_effort_yaw] -> Mixer/6(cmd_effort_yaw)
  PID Controller15/1 -> [m_ay_world_cmd]
  Sum8/1 -> PID Controller8/1
  [SYS_DIR_ALPHA] -> Mixer/14(dir_alpha)
  [sp_y] -> Sum9/1
  Sum15/1 -> PID Controller15/1
  Sum12/1 -> PID Controller12/1
  [m_cmd_effort_y] -> Sum15/1
  [SYS_LIM_THRUST] -> Mixer/23(max_thrust)
  [sp_z] -> Sum10/1
  [m_cmd_effort_z] -> Mixer/3(cmd_thrust_z)
  [SYS_MASS] -> Mixer/12(m)
  PID Controller10/1 -> [m_cmd_effort_z]
  [SYS_DIR_MOTOR_TOP] -> Mixer/22(dir_top)
  PID Controller9/1 -> [m_cmd_effort_y]
  [math_pitch] -> Sum12/2
  PID Controller13/1 -> [m_cmd_effort_yaw]
  [simscape_yaw] -> Mixer/7(yaw)
  [m_ay_world_cmd] -> Mixer/2(ay_world)
  [m_ax_world_cmd] -> Mixer/1(ax_world)
  [SYS_GRAVITY] -> Mixer/13(g)
  Sum11/1 -> PID Controller11/1
  [math_y] -> Sum9/2
  [SYS_COAX_TQ_EFF] -> Mixer/20(lam_c)
  [sp_pitch] -> Sum12/1
  [math_v] -> Memory10/1
  [m_phys_alpha] -> Memory5/1
  [SYS_COAX_EFF] -> Mixer/19(eta_c)
  [sp_roll] -> Sum11/1
  [sp_x] -> Sum8/1
  Memory9/1 -> Sum14/2
  Mixer/1(cmd_hw_alpha) -> [m_cmd_alpha]
  [math_roll] -> Sum11/2
  [simscape_roll] -> Mixer/9(roll)
  [SYS_KQ] -> Mixer/21(c_q)
  [math_z] -> Sum10/2
  Memory6/1 -> Mixer/11(phys_beta_hw)
  PID Controller8/1 -> [m_cmd_effort_x]
  Sum13/1 -> PID Controller13/1
  Memory5/1 -> Mixer/10(phys_alpha_hw)
  PID Controller14/1 -> [m_ax_world_cmd]
  Sum9/1 -> PID Controller9/1
  Demux12/2 -> [math_q]
  [math_attitude] -> Demux10/1
  Demux11/1 -> [math_u]
  Demux11/3 -> [math_w]
  [math_velocity] -> Demux11/1
  Demux10/2 -> [math_pitch]
  Demux12/1 -> [math_p]
  Demux12/3 -> [math_r]
  Demux1/1 -> [math_x]
  Gain1/1 -> [math_z]
  Demux10/1 -> [math_roll]
  [math_rate] -> Demux12/1
  [math_position] -> Demux1/1
  Demux1/2 -> [math_y]
  Demux1/3 -> Gain1/1
  Demux10/3 -> [math_yaw]
  Demux11/2 -> [math_v]
  PID Controller12/1 -> [m_cmd_effort_pitch]
  [m_cmd_effort_pitch] -> Mixer/5(cmd_effort_pitch)

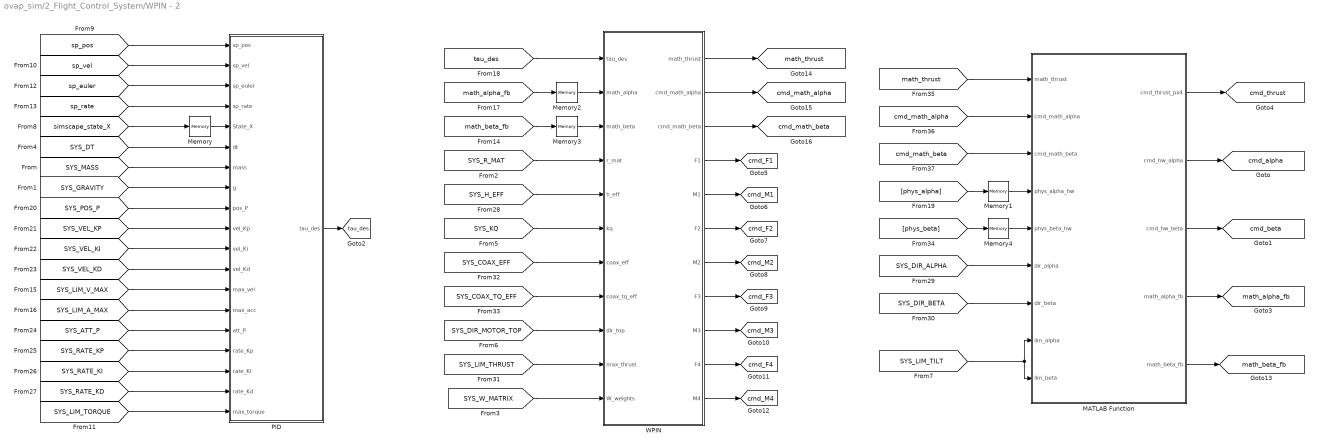
== system ovap_sim/2_Flight_Control_System/WPIN - 2 ==
  MATLAB Function : MATLAB Function  TreatAsAtomicUnit=on
  Memory{,1..4} (5 alike) : Memory
  PID : MATLAB Function  TreatAsAtomicUnit=on
  WPIN : MATLAB Function  TreatAsAtomicUnit=on
  tag scope: cmd_F1=global, cmd_F2=global, cmd_F3=global, cmd_F4=global, cmd_M1=global, cmd_M2=global, cmd_M3=global, cmd_M4=global, cmd_alpha=global, cmd_beta=global, cmd_math_alpha=global, cmd_math_beta=global, cmd_thrust=global, math_alpha_fb=global, math_beta_fb=global, math_thrust=global, tau_des=global
  wires:
  Memory/1 -> PID/5(State_X)
  [SYS_DIR_MOTOR_TOP] -> WPIN/9(dir_top)
  [SYS_RATE_KI] -> PID/17(rate_Ki)
  [SYS_VEL_KP] -> PID/10(vel_Kp)
  [SYS_MASS] -> PID/7(mass)
  [math_beta_fb] -> Memory3/1
  [SYS_LIM_TORQUE] -> PID/19(max_torque)
  [SYS_VEL_KI] -> PID/11(vel_Ki)
  [cmd_math_alpha] -> MATLAB Function/2(cmd_math_alpha)
  MATLAB Function/5(math_beta_fb) -> [math_beta_fb]
  [SYS_GRAVITY] -> PID/8(g)
  Memory4/1 -> MATLAB Function/5(phys_beta_hw)
  [SYS_KQ] -> WPIN/6(kq)
  [phys_alpha] -> Memory1/1
  WPIN/3(cmd_math_beta) -> [cmd_math_beta]
  [SYS_DIR_ALPHA] -> MATLAB Function/6(dir_alpha)
  MATLAB Function/3(cmd_hw_beta) -> [cmd_beta]
  WPIN/1(math_thrust) -> [math_thrust]
  MATLAB Function/2(cmd_hw_alpha) -> [cmd_alpha]
  [SYS_COAX_EFF] -> WPIN/7(coax_eff)
  WPIN/5(M1) -> [cmd_M1]
  [SYS_COAX_TQ_EFF] -> WPIN/8(coax_tq_eff)
  [SYS_H_EFF] -> WPIN/5(h_eff)
  [math_thrust] -> MATLAB Function/1(math_thrust)
  [tau_des] -> WPIN/1(tau_des)
  WPIN/9(M3) -> [cmd_M3]
  [SYS_LIM_THRUST] -> WPIN/10(max_thrust)
  [simscape_state_X] -> Memory/1
  [sp_pos] -> PID/1(sp_pos)
  [SYS_LIM_TILT] -> MATLAB Function/8(lim_alpha), MATLAB Function/9(lim_beta)
  [sp_euler] -> PID/3(sp_euler)
  [cmd_math_beta] -> MATLAB Function/3(cmd_math_beta)
  [SYS_LIM_A_MAX] -> PID/14(max_acc)
  WPIN/11(M4) -> [cmd_M4]
  Memory2/1 -> WPIN/2(math_alpha)
  [SYS_W_MATRIX] -> WPIN/11(W_weights)
  Memory3/1 -> WPIN/3(math_beta)
  WPIN/8(F3) -> [cmd_F3]
  WPIN/10(F4) -> [cmd_F4]
  [sp_vel] -> PID/2(sp_vel)
  WPIN/6(F2) -> [cmd_F2]
  [SYS_RATE_KD] -> PID/18(rate_Kd)
  [SYS_RATE_KP] -> PID/16(rate_Kp)
  [SYS_DT] -> PID/6(dt)
  PID/1(tau_des) -> [tau_des]
  [SYS_VEL_KD] -> PID/12(vel_Kd)
  MATLAB Function/4(math_alpha_fb) -> [math_alpha_fb]
  [phys_beta] -> Memory4/1
  [SYS_POS_P] -> PID/9(pos_P)
  [SYS_DIR_BETA] -> MATLAB Function/7(dir_beta)
  WPIN/7(M2) -> [cmd_M2]
  WPIN/4(F1) -> [cmd_F1]
  [sp_rate] -> PID/4(sp_rate)
  Memory1/1 -> MATLAB Function/4(phys_alpha_hw)
  [SYS_ATT_P] -> PID/15(att_P)
  WPIN/2(cmd_math_alpha) -> [cmd_math_alpha]
  [math_alpha_fb] -> Memory2/1
  [SYS_LIM_V_MAX] -> PID/13(max_vel)
  MATLAB Function/1(cmd_thrust_px4) -> [cmd_thrust]
  [SYS_R_MAT] -> WPIN/4(r_mat)

== matlab function ovap_sim/1_Mission_Planner/MATLAB Function ==
  settings: updateMethod=DISCRETE
  data: t input; dt input; v_max_lim input; a_max_lim input; w_max_lim input; ang_a_max_lim input; sp_pos output; sp_vel output; sp_acc output; sp_euler output; sp_rate output; tilt_lim input; sp_rate_dot output; tilt_rate_lim input; g_val input
function [sp_pos, sp_vel, sp_acc, sp_euler, sp_rate, sp_rate_dot] = Mission_Planner_Simulink(...
    t, ...
    dt, ...
    v_max_lim, ...      % Kết nối với SYS_LIM_V_MAX
    a_max_lim, ...      % Kết nối với SYS_LIM_A_MAX
    w_max_lim, ...      % Kết nối với SYS_LIM_W_MAX
    ang_a_max_lim, ...  % Kết nối với SYS_LIM_ANG_A_MAX
    tilt_lim, ...       % Kết nối với SYS_LIM_TILT (Góc bẻ ngàm tối đa)
    tilt_rate_lim, ...  % Kết nối với SYS_RATE_LIM_TILT (Tốc độ xoay servo)
    g_val)              % Hằng số trọng trường (9.81)

% =========================================================================
% BỘ QUY HOẠCH QUỸ ĐẠO TÍCH HỢP CHO SIMULINK (HỆ FRD)
% [CẬP NHẬT]: Sử dụng các biến rời rạc từ Workspace/Constant blocks
% =========================================================================

    % Khởi tạo bộ nhớ trạng thái quỹ đạo (Persistent)
    persistent traj
    if isempty(traj)
        traj.pos   = zeros(3,1); 
        traj.vel   = zeros(3,1); 
        traj.acc   = zeros(3,1);
        traj.euler = zeros(3,1); 
        traj.rate  = zeros(3,1); 
        traj.rate_dot = zeros(3,1);
    end

    % --- 1. MISSION MANAGER (Tạo mục tiêu theo thời gian) ---
    target_pos = [0; 0; 0];
    target_euler_deg = [0; 0; 0]; 
    planner_mode = 1;

    if t < 5.0
        target_pos = [0; 0; 5.0];        
    elseif t < 15.0
        target_pos = [0; 0; 5.0];       
        target_euler_deg = [0; 0; 0];   
    elseif t < 25.0
        target_pos = [0; 0; 10.0];     
        target_euler_deg = [0; 0; 0];  
    else
        target_pos = [0; 0; 10];        
        target_euler_deg = [70; 0; 0];
    end

    % Chuyển đổi đơn vị và chuẩn hóa Yaw
    target_euler = target_euler_deg * (pi / 180);
    target_euler(3) = atan2(sin(target_euler(3)), cos(target_euler(3)));

    % --- 2. MODE 0: STEP RESPONSE (Dùng để Tune PID) ---
    if planner_mode == 0
        sp_pos = target_pos; sp_vel = zeros(3,1); sp_acc = zeros(3,1);
        sp_euler = target_euler; sp_rate = zeros(3,1); sp_rate_dot = zeros(3,1);
        
        traj.pos = target_pos; traj.euler = target_euler;
        traj.vel = zeros(3,1); traj.rate = zeros(3,1);
        return;
    end

    % --- 3. TÍNH TOÁN RÀNG BUỘC PHẦN CỨNG (Anti-Saturation) ---
    % Gia tốc ngang tối đa dựa trên góc bẻ ngàm thực tế (SYS_LIM_TILT)
    a_max_hw_x = g_val * sin(tilt_lim);
    a_max_hw_y = g_val * sin(tilt_lim);
    
    % Jerk tối đa dựa trên tốc độ xoay thực tế của Servo (SYS_RATE_LIM_TILT)
    jerk_max_hw_x = g_val * tilt_rate_lim;
    jerk_max_hw_y = g_val * tilt_rate_lim;

    % --- 4. QUY HOẠCH VỊ TRÍ (XYZ) ---
    kp_pos = 1.5; 
    for i = 1:3
        pos_err = target_pos(i) - traj.pos(i);
        
        % Vận tốc mục tiêu (S-Curve bằng tanh)
        v_des = v_max_lim(i) * tanh((kp_pos * pos_err) / v_max_lim(i));
        
        % Tính toán Gia tốc (có chặn Jerk cho trục X, Y)
        a_needed = (v_des - traj.vel(i)) / dt;
        
        if i < 3 % Trục X và Y chịu ràng buộc Servo
            j_max = (i == 1) * jerk_max_hw_x + (i == 2) * jerk_max_hw_y;
            jerk_req = (a_needed - traj.acc(i)) / dt;
            jerk_req = max(min(jerk_req, j_max), -j_max);
            
            a_cmd = traj.acc(i) + jerk_req * dt;
            a_lim = (i == 1) * a_max_hw_x + (i == 2) * a_max_hw_y;
            a_cmd = max(min(a_cmd, min(a_max_lim(i), a_lim)), -min(a_max_lim(i), a_lim));
        else % Trục Z (Motor đáp ứng nhanh)
            a_cmd = max(min(a_needed, a_max_lim(i)), -a_max_lim(i));
        end
        
        % Tích phân
        traj.acc(i) = a_cmd;
        traj.vel(i) = traj.vel(i) + a_cmd * dt;
        traj.pos(i) = traj.pos(i) + traj.vel(i) * dt;
    end

    % --- 5. QUY HOẠCH TƯ THẾ (Euler) ---
    kp_att = 2.0;
    for k = 1:3
        % Xử lý Shortest Path cho Yaw
        if k == 3
            ang_err = atan2(sin(target_euler(k) - traj.euler(k)), ...
                            cos(target_euler(k) - traj.euler(k)));
        else
            ang_err = target_euler(k) - traj.euler(k);
        end
        
        % Vận tốc góc mục tiêu
        rate_des = w_max_lim(k) * tanh((kp_att * ang_err) / w_max_lim(k));
        
        % Gia tốc góc (sp_rate_dot)
        alpha_req = (rate_des - traj.rate(k)) / dt;
        alpha_cmd = max(min(alpha_req, ang_a_max_lim(k)), -ang_a_max_lim(k));
        
        % Tích phân
        traj.rate_dot(k) = alpha_cmd;
        traj.rate(k)     = traj.rate(k) + alpha_cmd * dt;
        traj.euler(k)    = traj.euler(k) + traj.rate(k) * dt;
    end

    % --- 6. XUẤT TÍN HIỆU ĐẦU RA ---
    sp_pos      = traj.pos;
    sp_vel      = traj.vel;
    sp_acc      = traj.acc;
    sp_euler    = traj.euler;
    sp_rate     = traj.rate;
    sp_rate_dot = traj.rate_dot;
end

== matlab function ovap_sim/3_Actuator_Dynamics/MATLAB Function ==
  settings: updateMethod=DISCRETE  sampleTime=0.002
  data: cmd_thrust input; phys_thrust output; cmd_alpha input; cmd_beta input; dt input; tau_motor input; tau_servo input; rate_lim input; lim_tilt input; phys_alpha output; phys_beta output
function [phys_thrust, phys_alpha, phys_beta] = Actuator_Dynamics(cmd_thrust, cmd_alpha, cmd_beta, ...
    dt, tau_motor, tau_servo, rate_lim, lim_tilt)
% =========================================================================
% Tên hàm: Actuator_Dynamics (Động lực học Cơ cấu chấp hành)
% Chức năng: Đóng vai trò làm "Bộ lọc Hiện thực". Biến các mệnh lệnh toán học
%            tức thời (cmd_) thành phản ứng vật lý thực tế có độ trễ (phys_).
% Nguyên lý: Mô phỏng Quán tính Rotor (First-Order Lag) và Giới hạn bánh răng
%            Servo (Rate Limit & Saturation).
% =========================================================================

    % ---------------------------------------------------------------------
    % 1. BỘ NHỚ VẬT LÝ (PERSISTENT STATE)
    % Ý nghĩa: Trong thế giới thực, một vật thể không thể dịch chuyển tức thời
    % từ trạng thái A sang B. Trạng thái tiếp theo luôn phụ thuộc vào trạng
    % thái hiện tại. Biến persistent đóng vai trò là "quán tính" của hệ thống.
    % ---------------------------------------------------------------------
    persistent prev_thrust prev_alpha prev_beta
    
    % Khởi tạo trạng thái đứng im khi bắt đầu bật điện (t = 0)
    if isempty(prev_thrust)
        prev_thrust = zeros(8,1); % Lực đẩy 8 motor = 0 N
        prev_alpha  = zeros(4,1); % Góc gật 4 ngàm = 0 rad
        prev_beta   = zeros(4,1); % Góc lật 4 ngàm = 0 rad
    end

    % ---------------------------------------------------------------------
    % 2. ĐỘNG LỰC HỌC ĐỘNG CƠ (MOTOR DYNAMICS - THUẬT TOÁN PT1)
    % Bản chất: Lõi chuông motor và cánh quạt 7-inch có khối lượng (Inertia).
    % Khi ESC bơm dòng điện, từ trường sinh ra momen xoắn để thắng sức ỳ này.
    % Thời gian để đạt được lực đẩy yêu cầu được đặc trưng bởi tau_motor (Ví dụ: 0.03s).
    % ---------------------------------------------------------------------
    % Tính hệ số lọc (Alpha) của bộ lọc thông thấp bậc 1 (First-Order Low-pass)
    % Hệ số này quyết định motor "bám theo" lệnh nhanh hay chậm dựa trên bước nhảy dt.
    alpha_m = dt / (tau_motor + dt);
    
    % Lực đẩy thực tế sẽ bám đuổi (chasing) lệnh yêu cầu.
    % Nếu lệch càng nhiều (cmd - prev lớn), motor tăng tốc càng mạnh.
    thrust_next = prev_thrust + alpha_m * (cmd_thrust - prev_thrust);
    
    % Giới hạn vật lý: Động cơ BLDC gắn cánh quạt tĩnh không thể tạo lực đẩy âm
    % (Trừ khi ESC dùng chế độ 3D đảo chiều quay, nhưng OVAP-X1 không dùng).
    phys_thrust = max(0, thrust_next); 

    % ---------------------------------------------------------------------
    % 3. ĐỘNG LỰC HỌC SERVO (SERVO DYNAMICS - LAG & RATE LIMIT)
    % Bản chất: Servo xịn như KST có mạch điều khiển bên trong (gây trễ tau_servo),
    % và hộp số bánh răng kim loại có tốc độ quay tối đa (rate_lim, ví dụ: 300 deg/s).
    % ---------------------------------------------------------------------
    % Hệ số độ trễ của mạch điện điều khiển Servo
    alpha_s = dt / (tau_servo + dt);
    
    % GIỚI HẠN TỐC ĐỘ (Rate Limit): Quãng đường góc lớn nhất (rad) mà bánh răng 
    % cơ khí có thể quét được trong khoảng thời gian siêu ngắn dt (0.002s).
    max_step = rate_lim * dt; 
    
    % ================= KÊNH ALPHA (NGÀM GẬP PITCH) =================
    % 3.1. Tính vị trí lý tưởng mà Servo "muốn" đạt tới (chỉ xét độ trễ mạch điện)
    ideal_alpha = prev_alpha + alpha_s * (cmd_alpha - prev_alpha); 
    
    % 3.2. Tính quãng đường góc cần di chuyển trong bước này
    delta_alpha = ideal_alpha - prev_alpha;
    
    % 3.3. ÁP DỤNG NÚT THẮT CỔ CHAI CƠ KHÍ (Rate Clamping)
    % Nếu lệnh bắt Servo quay nhanh hơn khả năng của motor bên trong, 
    % nó sẽ bị "nghẽn" lại và chỉ xoay được đúng bằng max_step.
    delta_alpha = max(min(delta_alpha, max_step), -max_step);      
    
    % 3.4. Vị trí thực tế Servo đạt được sau 1 bước dt
    phys_alpha = prev_alpha + delta_alpha;
    
    % 3.5. VA CHẠM CƠ KHÍ (Hard Stop / Saturation)
    phys_alpha = max(min(phys_alpha, lim_tilt), -lim_tilt);        
    
    % ================= KÊNH BETA (NGÀM LẬT ROLL) =================
    % (Áp dụng chính xác các quy luật vật lý tương tự như Kênh Alpha)
    ideal_beta = prev_beta + alpha_s * (cmd_beta - prev_beta);     
    delta_beta = ideal_beta - prev_beta;
    delta_beta = max(min(delta_beta, max_step), -max_step);        
    
    phys_beta = prev_beta + delta_beta;
    phys_beta = max(min(phys_beta, lim_tilt), -lim_tilt);          

    % ---------------------------------------------------------------------
    % 4. CẬP NHẬT TRẠNG THÁI (TIME MARCHING)
    % Ý nghĩa: Dòng thời gian trôi đi. Hiện tại của vòng lặp này sẽ trở thành 
    % quá khứ (prev_) cho vòng lặp tích phân tiếp theo.
    % ---------------------------------------------------------------------
    prev_thrust = phys_thrust;
    prev_alpha  = phys_alpha;
    prev_beta   = phys_beta;
end
